simulink model "MoPhongCoDieuKhien"  (R2022b)
settings: Solver=FixedStepAuto  StartTime=0.0  StopTime=100  FixedStep=0.01  RelTol=1e-3
values from neighbouring files (symbols this model uses):
  l = 0.5    [ThongSo.m]
  M = 1    [ThongSo.m]
  m = 0.1    [ThongSo.m]
settings Model: Creator=vanph  LastModifiedBy=vanph

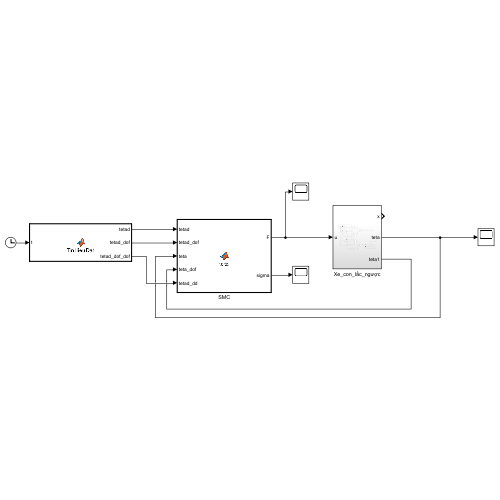
[thumbnail: Simulink's stored preview of the top-level diagram]
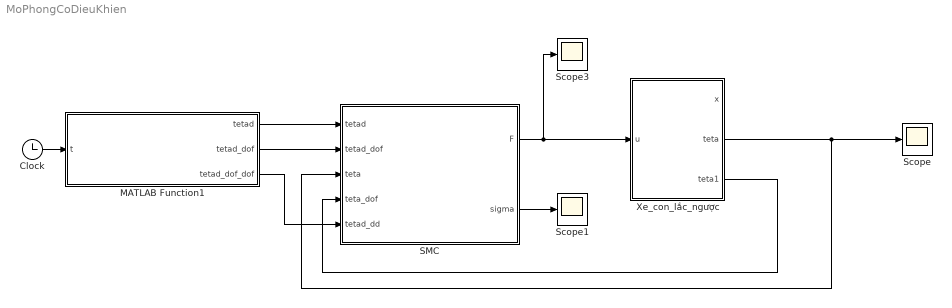
== system MoPhongCoDieuKhien ==
  Clock : Clock
      settings: Decimation=100
  MATLAB Function1 : MATLAB Function  TreatAsAtomicUnit=on
  SMC : MATLAB Function  TreatAsAtomicUnit=on
  Scope : Scope
  Scope1 : Scope
  Scope3 : Scope
  Xe_con_lắc_ngược : Subsystem
  wires:
  Xe_con_lắc_ngược/2(teta) -> Scope/1, SMC/3(teta)
  SMC/1(F) -> Scope3/1, Xe_con_lắc_ngược/1(u)
  Xe_con_lắc_ngược/3(teta1) -> SMC/4(teta_dof)
  MATLAB Function1/1(tetad) -> SMC/1(tetad)
  MATLAB Function1/2(tetad_dof) -> SMC/2(tetad_dof)
  Clock/1 -> MATLAB Function1/1(t)
  SMC/2(sigma) -> Scope1/1
  MATLAB Function1/3(tetad_dof_dof) -> SMC/5(tetad_dd)

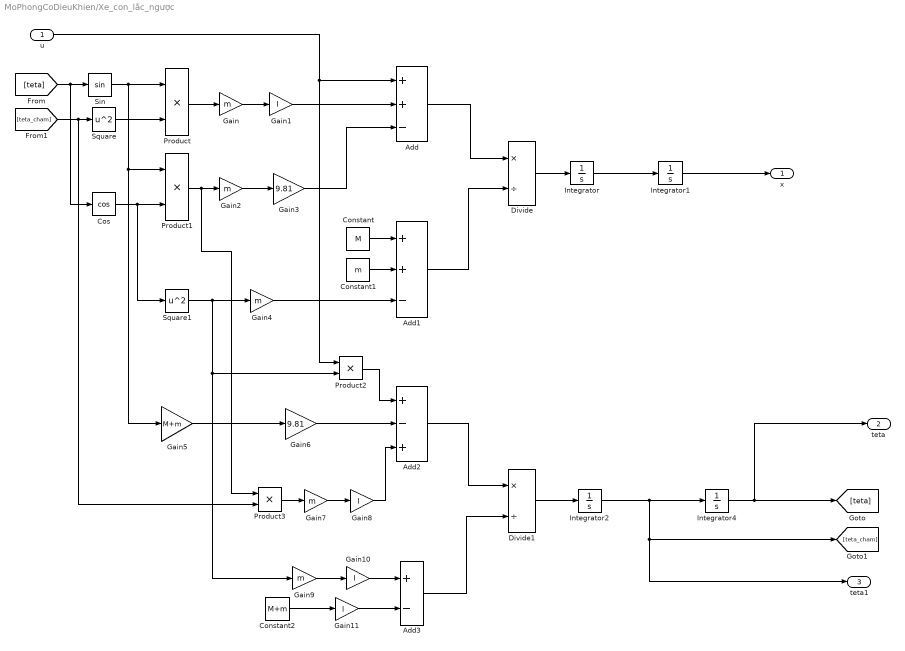
== system MoPhongCoDieuKhien/Xe_con_lắc_ngược ==
  u : Inport
  Add : Sum  Inputs=++-
  Add1 : Sum  Inputs=++-
  Add2 : Sum  Inputs=+-+
  Add3 : Sum  Inputs=+-
  Constant : Constant  Value=M
  Constant1 : Constant  Value=m
  Constant2 : Constant  Value=M+m
  Cos : Trigonometry  Operator=cos
  Divide : Product  Inputs=*/
  Divide1 : Product  Inputs=*/
  Gain{,2,4,7,9} (5 alike) : Gain  Gain=m
  Gain{1,8,10..11} (4 alike) : Gain  Gain=l
  Gain3 : Gain  Gain=9.81
  Gain5 : Gain  Gain=M+m
  Gain6 : Gain  Gain=9.81
  Integrator : Integrator
  Integrator1 : Integrator
  Integrator2 : Integrator
  Integrator4 : Integrator  InitialCondition=1
  Product{,1..3} (4 alike) : Product
  Sin : Trigonometry
  Square : Math  Operator=square
  Square1 : Math  Operator=square
  x : Outport
  teta : Outport  Port=2
  teta1 : Outport  Port=3
  wires:
  Add1/1 -> Divide/2
  Product3/1 -> Gain7/1
  Gain3/1 -> Add/3
  Gain6/1 -> Add2/2
  Cos/1 -> Square1/1, Product1/2
  Gain4/1 -> Add1/3
  Add2/1 -> Divide1/1
  [teta_cham] -> Product3/2, Square/1
  Gain7/1 -> Gain8/1
  Product1/1 -> Product3/1, Gain2/1
  Constant/1 -> Add1/1
  Gain10/1 -> Add3/1
  Constant2/1 -> Gain11/1
  [teta] -> Cos/1, Sin/1
  Sin/1 -> Gain5/1, Product1/1, Product/1
  Integrator/1 -> Integrator1/1
  Gain/1 -> Gain1/1
  Product2/1 -> Add2/1
  Add3/1 -> Divide1/2
  Integrator4/1 -> [teta], teta/1
  Gain8/1 -> Add2/3
  Gain2/1 -> Gain3/1
  Square1/1 -> Gain9/1, Product2/2, Gain4/1
  Gain9/1 -> Gain10/1
  Square/1 -> Product/2
  u/1 -> Add/1, Product2/1
  Product/1 -> Gain/1
  Gain5/1 -> Gain6/1
  Gain1/1 -> Add/2
  Divide/1 -> Integrator/1
  Integrator1/1 -> x/1
  Gain11/1 -> Add3/2
  Constant1/1 -> Add1/2
  Add/1 -> Divide/1
  Divide1/1 -> Integrator2/1
  Integrator2/1 -> teta1/1, [teta_cham], Integrator4/1

== matlab function MoPhongCoDieuKhien/MATLAB Function1 ==
  data: t input; tetad output; tetad_dof output; tetad_dof_dof output
function [tetad, tetad_dof, tetad_dof_dof] = TinHieuDat(t)

tetad = 0*sin(t);
tetad_dof = 0*sin(t);
tetad_dof_dof = 0*sin(t);

== matlab function MoPhongCoDieuKhien/SMC ==
  data: tetad input; F output; tetad_dof input; teta input; teta_dof input; sigma output; tetad_dd input
function [F, sigma] = teta(tetad, tetad_dof, teta, teta_dof, tetad_dd)

m = 0.1;
l = 0.5;
M = 1;
g = 9.81;
lamda = 20;
K = 5;
eta = 5;
e = teta - tetad;
e_d = teta_dof - tetad_dof;
sigma = lamda*e + e_d;

f_k = (-(M+m)*g*sin(teta)+m*l*cos(teta)*sin(teta)*teta_dof^2)/(m*l*cos(teta)^2-(M+m)*l);
g_k = (cos(teta))/(m*l*cos(teta)^2-(M+m)*l);

F = -(1/g_k)*(f_k+K*sigma+lamda*e_d+eta*sign(sigma)-tetad_dd);
